simulink model "downlink_4c2t"  (Simulink 8.7)
settings: Solver=VariableStepDiscrete  StartTime=0.0  StopTime=DUC_LINEUP_param.endTime  RelTol=1e-3
PreLoadFcn:
  | % Run the setup script when the model is opened
  | setup_downlink_4c2t;
InitFcn:
  | % Run the setup script again just before the
  | % model is run, so that any updates made
  | % after opening are applied.
  | setup_downlink_4c2t;
  | 
  | %% DSPBuilder Start
  | alt_dspbuilder_update_model(bdroot)
  | %% DSPBuilder End
values from neighbouring files (symbols this model uses):
  LUTS_DPD_CLIP =     [downlink_4c2t_dpd_clip.mat]
  PulsExtention = 128    [setup_downlink_4c2t.m]
  StartAddress1 = Iter1_Param.BaseAddr + 3200    [setup_downlink_4c2t.m]
  StartAddress2 = StartAddress1+1024    [setup_downlink_4c2t.m]
  win = [w(1:PulsExtention) ones(1,Iter0_Param.pulseLen) w(PulsExtention+1:end)]    [setup_downlink_4c2t.m]
undefined symbols (not defined in the file or in its folder): AdvDSPBChannelOutDisplay, AdvDSPBDMemDisplay, dpoly, dspba_ChannelInVis, dspba_ChannelOutVis, dspba_internal_get_channel_ports, dspba_internal_get_demux_ports, DUC_LINEUP_param, evalAionMaskParam, iq_width, Iter0_Param, latency, primtype, REG, UseDontCare, value
undefined symbols (not defined in the file): cfr0_id, cfr_Params0, cfr_Params1, clock_rate, REG_dut_id_addr
libraries: DSPBAPrim x1438, DSPBAControl x77, DSPBAModelBus x71, DSPBABase x40, downlink_4c2t_foldingcfr_3firs_lib x26, DSPBAUtilities x8, downlink_4c2t_lib x4, downlink_4c2t_cordic_lib x2, downlink_4c2t_dpd_clipper x2, DSPBAFilters x2, DSPBAWaveformSynth x2, downlink_4c2t_lduc_lib x1
(part 2 of 17)

== system downlink_4c2t/DUT/COMPLEX_REAL ==
  a1 : Inport
  v : Inport  Port=2
  c : Inport  Port=3
  ChannelIn : DSPBAPrim/ChannelIn  primtype=channelin  nInputs=dspba_internal_get_channel_ports(gcb)  nOutputs=dspba_internal_get_channel_ports(gcb)  omode=Inherit via internal rule  otype=sfix(16)  scale=2^-15  rndmethod=Unbiased  factor=1  satmethod=Symmetric  shift_vec=[0 1 2 -1]  value=1  inPortNames=['v'; 'c'; '0'; '1'; '2'; '3'; '4'; '5'; '6'; '7'; '8'; '9'; 'A'; 'B'; 'D'; 'E'; 'F'; 'G'; 'H'; 'I'; 'J'; 'K'; 'L'; 'M'; 'N'; 'O'; 'P'; 'Q'; 'R'; 'S'; 'T'; 'U'; 'W'; 'X'; 'Y'; 'Z']  outPortNames=['v'; 'c'; '0'; '1'; '2'; '3'; '4'; '5'; '6'; '7'; '8'; '9'; 'A'; 'B'; 'D'; 'E'; 'F'; 'G'; 'H'; 'I'; 'J'; 'K'; 'L'; 'M'; 'N'; 'O'; 'P'; 'Q'; 'R'; 'S'; 'T'; 'U'; 'W'; 'X'; 'Y'; 'Z']  dspbaimage=dspba_prim.jpg  text=fprintf('In');  style=Optimised  dataSignals=1  foldingEnabled=off  channels=1  sampleRate=200  packetBeginPresent=off  packetBeginEnabled=off  visibilities=dspba_ChannelInVis(gcb)  latencyCorrection=0  version=20141013
  ChannelOut : DSPBAPrim/ChannelOut  primtype=channelout  nInputs=dspba_internal_get_channel_ports(gcb)  nOutputs=dspba_internal_get_channel_ports(gcb)  omode=Inherit via internal rule  otype=sfix(16)  scale=2^-15  rndmethod=Unbiased  factor=1  satmethod=Symmetric  shift_vec=[0 1 2 -1]  value=4  inPortNames=['v'; 'c'; '0'; '1'; '2'; '3'; '4'; '5'; '6'; '7'; '8'; '9'; 'A'; 'B'; 'D'; 'E'; 'F'; 'G'; 'H'; 'I'; 'J'; 'K'; 'L'; 'M'; 'N'; 'O'; 'P'; 'Q'; 'R'; 'S'; 'T'; 'U'; 'W'; 'X'; 'Y'; 'Z']  outPortNames=['v'; 'c'; '0'; '1'; '2'; '3'; '4'; '5'; '6'; '7'; '8'; '9'; 'A'; 'B'; 'D'; 'E'; 'F'; 'G'; 'H'; 'I'; 'J'; 'K'; 'L'; 'M'; 'N'; 'O'; 'P'; 'Q'; 'R'; 'S'; 'T'; 'U'; 'W'; 'X'; 'Y'; 'Z']  dspbaimage=dspba_prim.jpg  text=fprintf('Out%s', AdvDSPBChannelOutDisplay(latency));  style=Optimised  dataSignals=4  foldingEnabled=off  channels=1  sampleRate=200  packetBeginPresent=off  packetBeginEnabled=off  visibilities=dspba_ChannelOutVis(gcb)  latency=0  latencyCorrection=0  version=20141013
  Complex to Real-Imag : ComplexToRealImag
  Complex to Real-Imag1 : ComplexToRealImag
  Const : DSPBAPrim/Const  primtype=const  nInputs=0  nOutputs=1  omode=Inherit via internal rule  otype=sfix(16)  scale=2^-15  rndmethod=Unbiased  factor=1  satmethod=Symmetric  shift_vec=[0 1 2 -1]  value=0  inPortNames=['+'; '+';]  outPortNames=[' ']  dspbaimage=dspba_prim.jpg  text=fprintf('%s', num2str(value));  style=Optimised  visibilities=8 + 1024  floatPrecision=float32_m23  version=20120820
  Demux4 : Demux  Outputs=2
  LocalThreshold : DSPBABase/LocalThreshold  margin=DUC_LINEUP_param.ClockMargin  delayRegOrRAMThresholdBits=-1  MediumDualMemThresholdBits=-1  LargeDualMemThresholdBits=-1  hardMultiplierThresholdLuts=-1  complexMultKaratsuba=off  version=0
  Mux : Mux
  SynthesisInfo : DSPBAPrim/SynthesisInfo  primtype=synthinfo  nInputs=0  nOutputs=0  omode=Inherit via internal rule  otype=sfix(16)  scale=2^-15  rndmethod=Truncate  factor=1  satmethod=Symmetric  shift_vec=[0 1 2 -1]  value=99  inPortNames=[' '; ' ';]  outPortNames=[' ']  dspbaimage=dspba_prim_ctrl.jpg  text=fprintf('Style=%s', style);  style=Scheduled  visibilities=2^15+2^17+2^18+2^19  constraintInUse=off  constraintRelation=>  constraintLimit=20  bitAccurate=off  version=20150220
  Terminator17 : Terminator
  q1 : Outport
  q_v : Outport  Port=2
  q_c : Outport  Port=3
  wires:
  ChannelIn/2 -> Terminator17/1
  Const/1 -> ChannelOut/2
  ChannelIn/1 -> ChannelOut/1
  ChannelIn/3 -> Demux4/1
  ChannelOut/2 -> q_c/1
  ChannelOut/1 -> q_v/1
  c/1 -> ChannelIn/2
  v/1 -> ChannelIn/1
  a1/1 -> ChannelIn/3
  Demux4/1 -> Complex to Real-Imag/1
  Demux4/2 -> Complex to Real-Imag1/1
  Complex to Real-Imag/1 -> ChannelOut/3
  Complex to Real-Imag/2 -> ChannelOut/4
  Complex to Real-Imag1/1 -> ChannelOut/5
  Complex to Real-Imag1/2 -> ChannelOut/6
  ChannelOut/3 -> Mux/1
  ChannelOut/4 -> Mux/2
  Mux/1 -> q1/1
  ChannelOut/5 -> Mux/3
  ChannelOut/6 -> Mux/4

== system downlink_4c2t/DUT/DPD ==
  dpd_ant1_data : Inport
  dpd_ant2_data : Inport  Port=2
  sink_valid : Inport  Port=3
  sink_channel : Inport  Port=4
  Const{1..6} (6 alike) : DSPBAPrim/Const  primtype=const  nInputs=0  nOutputs=1  omode=Inherit via internal rule  otype=sfix(16)  scale=2^-15  rndmethod=Unbiased  factor=1  satmethod=Symmetric  shift_vec=[0 1 2 -1]  value=0  inPortNames=['+'; '+';]  outPortNames=[' ']  dspbaimage=dspba_prim.jpg  text=fprintf('%s', num2str(value));  style=Optimised  visibilities=8 + 1024  floatPrecision=float32_m23  version=20120820
  DPD_ANT1 : Subsystem
  DPD_ANT2 : Subsystem
  Terminator{,1..3} (4 alike) : Terminator
  complex_real_converter : Subsystem
  complex_real_converter1 : Subsystem
  source_data : Outport
  source_valid : Outport  Port=2
  source_channel : Outport  Port=3
  source_data1 : Outport  Port=4
  source_valid1 : Outport  Port=5
  source_channel1 : Outport  Port=6
  wires:
  DPD_ANT1/1(v) -> source_valid/1
  DPD_ANT1/2(c) -> source_channel/1
  Const5/1 -> DPD_ANT1/4(sop)
  Const3/1 -> DPD_ANT1/5(eop)
  Const1/1 -> DPD_ANT1/6(Arb)
  DPD_ANT1/4(sop_out) -> Terminator/1
  DPD_ANT1/5(eop_out) -> Terminator1/1
  DPD_ANT2/2(c) -> source_channel1/1
  Const6/1 -> DPD_ANT2/4(sop)
  Const4/1 -> DPD_ANT2/5(eop)
  Const2/1 -> DPD_ANT2/6(Arb)
  DPD_ANT2/4(sop_out) -> Terminator2/1
  DPD_ANT2/5(eop_out) -> Terminator3/1
  sink_channel/1 -> DPD_ANT2/2(channel), DPD_ANT1/2(channel)
  sink_valid/1 -> DPD_ANT2/1(valid), DPD_ANT1/1(valid)
  DPD_ANT2/1(v) -> source_valid1/1
  dpd_ant1_data/1 -> DPD_ANT1/3(xr)
  dpd_ant2_data/1 -> DPD_ANT2/3(xr)
  DPD_ANT1/3(zr) -> complex_real_converter/1(In1)
  complex_real_converter/1(Out1) -> source_data/1
  DPD_ANT2/3(zr) -> complex_real_converter1/1(In1)
  complex_real_converter1/1(Out1) -> source_data1/1

== system downlink_4c2t/DUT/DPD1_CLIPPER ==
  "data " : Inport
  valid : Inport  Port=2
  channel : Inport  Port=3
  scale_bit : Inport  Port=4
  Demux : Demux  Outputs=2
  Scale : DSPBABase/Scale  otype=sfix(16)  scale=2^-15  rndmethod=Unbiased  factor=1  satmethod=Symmetric  shift_vec=[0 1]  latency=9  wideSimulation=off  version=20130807
  Subsystem : Subsystem
  Terminator : Terminator
  bit_combine : downlink_4c2t_dpd_clipper/DPD_CLIPER/Subsystem/complex_real_converter
  DATA_Out : Outport
  Valid_Out : Outport  Port=2
  Chann_Out : Outport  Port=3
  wires:
  bit_combine/1 -> DATA_Out/1
  Scale/1 -> Demux/1
  Demux/1 -> bit_combine/1
  Demux/2 -> bit_combine/2
  Scale/2 -> Valid_Out/1
  Scale/3 -> Chann_Out/1
  scale_bit/1 -> Scale/4
  Scale/4 -> Terminator/1
  Subsystem/1("data_out ") -> Scale/1
  Subsystem/2(valid_out) -> Scale/2
  Subsystem/3(channel_out) -> Scale/3
  "data "/1 -> Subsystem/1(data 1)
  valid/1 -> Subsystem/2(valid1)
  channel/1 -> Subsystem/3(channel1)

== system downlink_4c2t/DUT/DPD2_CLIPPER ==
  "data " : Inport
  valid : Inport  Port=2
  channel : Inport  Port=3
  scale_bit : Inport  Port=4
  Demux : Demux  Outputs=2
  Scale : DSPBABase/Scale  otype=sfix(16)  scale=2^-15  rndmethod=Unbiased  factor=1  satmethod=Symmetric  shift_vec=[0 1]  latency=9  wideSimulation=off  version=20130807
  Subsystem : Subsystem
  Terminator : Terminator
  bit_combine : downlink_4c2t_dpd_clipper/DPD_CLIPER/Subsystem/complex_real_converter
  DATA_Out : Outport
  Valid_Out : Outport  Port=2
  Chann_Out : Outport  Port=3
  wires:
  channel/1 -> Subsystem/3(channel1)
  valid/1 -> Subsystem/2(valid1)
  "data "/1 -> Subsystem/1(data 1)
  Subsystem/3(channel_out) -> Scale/3
  Subsystem/2(valid_out) -> Scale/2
  Subsystem/1("data_out ") -> Scale/1
  Scale/4 -> Terminator/1
  scale_bit/1 -> Scale/4
  Scale/3 -> Chann_Out/1
  Scale/2 -> Valid_Out/1
  Demux/2 -> bit_combine/2
  Demux/1 -> bit_combine/1
  Scale/1 -> Demux/1
  bit_combine/1 -> DATA_Out/1

== system downlink_4c2t/DUT/DPD_ANT1_IN_rfp ==
  GPOut : DSPBAPrim/GPOut  primtype=gpout  nInputs=evalAionMaskParam(gcb,'value',1)  nOutputs=evalAionMaskParam(gcb,'value',1)  omode=Inherit via internal rule  otype=sfix(16)  scale=2^-15  rndmethod=Unbiased  factor=1  satmethod=Symmetric  shift_vec=[0 1 2 -1]  value=1  inPortNames=[' ' ' ' ' ' ' ' ' ' ' ' ' ' ' ' ' ' ' ' ' ' ' ' ' ' ' ' ' ' ' ' ' ' ' ' ' ' ' ' ' ' ' ' ' ' ' ' ' ' ' ' ' ' ' ' ' ' ' ' ' ' ' ' ' ' ' ' ' ']'  outPortNames=[' ' ' ' ' ' ' ' ' ' ' ' ' ' ' ' ' ' ' ' ' ' ' ' ' ' ' ' ' ' ' ' ' ' ' ' ' ' ' ' ' ' ' ' ' ' ' ' ' ' ' ' ' ' ' ' ' ' ' ' ' ' ' ' ' ' ' ' ' ']'  dspbaimage=dspba_prim.jpg  text=fprintf('GPOut');  style=Optimised  visibilities=1024  latencyCorrection=0  version=20090407
  SynthesisInfo : DSPBAPrim/SynthesisInfo  primtype=synthinfo  nInputs=0  nOutputs=0  omode=Inherit via internal rule  otype=sfix(16)  scale=2^-15  rndmethod=Truncate  factor=1  satmethod=Symmetric  shift_vec=[0 1 2 -1]  value=99  inPortNames=[' '; ' ';]  outPortNames=[' ']  dspbaimage=dspba_prim_ctrl.jpg  text=fprintf('Style=%s', style);  style=Scheduled  visibilities=2^15+2^17+2^18+2^19  constraintInUse=off  constraintRelation=>  constraintLimit=2  bitAccurate=off  version=20150220
  zero_idx1 : DSPBAPrim/Const  primtype=const  nInputs=0  nOutputs=1  omode=boolean  otype=ufix(1)  scale=0  rndmethod=Unbiased  factor=1  satmethod=Symmetric  shift_vec=[0 1 2 -1]  value=1  inPortNames=['+'; '+';]  outPortNames=[' ']  dspbaimage=dspba_prim.jpg  text=fprintf('%s', num2str(value));  style=Optimised  visibilities=8 + 1024  floatPrecision=float32_m23  version=20120820
  Out_RFP : Outport
  wires:
  GPOut/1 -> Out_RFP/1
  zero_idx1/1 -> GPOut/1

== system downlink_4c2t/DUT/DUC_DPD1_OUT_PM ==
  note: I^2 + Q^2
  valid : Inport
  channel : Inport  Port=2
  "data " : Inport  Port=3
  pulse_1msec : Inport  Port=4
  Reg_busy_bit : Inport  Port=5
  Ant1_accumulator : Subsystem
  Ant1_peak_dedector : Subsystem
  BitExtract : DSPBAPrim/BitExtract  primtype=bitextract  nInputs=1  nOutputs=1  omode=Specify via dialog  otype=ufix(32)  scale=2^0  rndmethod=Unbiased  factor=1  satmethod=Symmetric  shift_vec=[0 1 2 -1]  value=0  inPortNames=[' '; ' ';]  outPortNames=[' ']  dspbaimage=dspba_prim.jpg  text=fprintf('..%d', value);  style=Optimised  visibilities=8+1024  version=20090407
  BitExtract1 : DSPBAPrim/BitExtract  primtype=bitextract  nInputs=1  nOutputs=1  omode=Specify via dialog  otype=ufix(32)  scale=2^0  rndmethod=Unbiased  factor=1  satmethod=Symmetric  shift_vec=[0 1 2 -1]  value=32  inPortNames=[' '; ' ';]  outPortNames=[' ']  dspbaimage=dspba_prim.jpg  text=fprintf('..%d', value);  style=Optimised  visibilities=8+1024  version=20090407
  Carr1_Accumulater1 : DSPBAModelBus/RegOut  reg_name=power_meter_param.dpd1_out_acc1_reg_addr  reg_rwmode=Read  reg_msb=31  reg_lsb=0  reg_desc=Description of what is stored in this register  reg_addr=9681  SampleTime=-1  version=20090407
  Carr1_Accumulater2 : DSPBAModelBus/RegOut  reg_name=power_meter_param.dpd1_out_acc2_reg_addr  reg_rwmode=Read  reg_msb=31  reg_lsb=0  reg_desc=Description of what is stored in this register  reg_addr=9682  SampleTime=-1  version=20090407
  Carr1_PD : DSPBAModelBus/RegOut  reg_name=power_meter_param.dpd1_out_pd_address  reg_rwmode=Read  reg_msb=31  reg_lsb=0  reg_desc=Description of what is stored in this register  reg_addr=9680  SampleTime=-1  version=20090407
  Const : DSPBAPrim/Const  primtype=const  nInputs=0  nOutputs=1  omode=Inherit via internal rule  otype=sfix(16)  scale=2^-15  rndmethod=Unbiased  factor=1  satmethod=Symmetric  shift_vec=[0 1 2 -1]  value=0  inPortNames=['+'; '+';]  outPortNames=[' ']  dspbaimage=dspba_prim.jpg  text=fprintf('%s', num2str(value));  style=Optimised  visibilities=8 + 1024  floatPrecision=float32_m23  version=20120820
  Edge_deductor : Subsystem
  Scale : DSPBABase/Scale  otype=sfix(16)  scale=2^-15  rndmethod=Unbiased  factor=1  satmethod=Symmetric  shift_vec=0  latency=6  wideSimulation=off  version=20130807
  Terminator1 : Terminator
  carrier_separation : Subsystem
  wires:
  BitExtract1/1 -> Carr1_Accumulater2/1
  BitExtract/1 -> Carr1_Accumulater1/1
  carrier_separation/3(channel_out) -> Scale/3
  carrier_separation/2(valid_out) -> Scale/2
  pulse_1msec/1 -> carrier_separation/4("1ms_pulse_in ")
  Scale/4 -> Terminator1/1
  "data "/1 -> carrier_separation/3("data ")
  channel/1 -> carrier_separation/2(channel)
  valid/1 -> carrier_separation/1(valid)
  Scale/2 -> Ant1_accumulator/2(valid1), Ant1_peak_dedector/2(valid)
  Scale/3 -> Ant1_accumulator/3(channel1), Ant1_peak_dedector/3(channel)
  Const/1 -> Scale/4
  carrier_separation/1("axc1_data_out ") -> Scale/1
  Scale/1 -> Ant1_accumulator/1(data), Ant1_peak_dedector/1(data_in)
  carrier_separation/4(pulse_1ms_out) -> Ant1_peak_dedector/4(pulse_1ms), Ant1_accumulator/4(pulse_1ms)
  Ant1_peak_dedector/1(Out_data) -> Carr1_PD/1
  Edge_deductor/1(Out1) -> Carr1_Accumulater2/2, Carr1_Accumulater1/2, Carr1_PD/2
  Ant1_peak_dedector/2(pulse_1ms_out) -> Edge_deductor/2(In2)
  Reg_busy_bit/1 -> Edge_deductor/1(In1)
  Ant1_accumulator/1(Out_data) -> BitExtract/1, BitExtract1/1

== system downlink_4c2t/DUT/DUC_DPD2_OUT_PM ==
  note: I^2 + Q^2
  valid : Inport
  channel : Inport  Port=2
  "data " : Inport  Port=3
  pulse_1msec : Inport  Port=4
  Reg_busy_bit : Inport  Port=5
  Ant1_accumulator : Subsystem
  Ant1_peak_dedector : Subsystem
  BitExtract : DSPBAPrim/BitExtract  primtype=bitextract  nInputs=1  nOutputs=1  omode=Specify via dialog  otype=ufix(32)  scale=2^0  rndmethod=Unbiased  factor=1  satmethod=Symmetric  shift_vec=[0 1 2 -1]  value=0  inPortNames=[' '; ' ';]  outPortNames=[' ']  dspbaimage=dspba_prim.jpg  text=fprintf('..%d', value);  style=Optimised  visibilities=8+1024  version=20090407
  BitExtract1 : DSPBAPrim/BitExtract  primtype=bitextract  nInputs=1  nOutputs=1  omode=Specify via dialog  otype=ufix(32)  scale=2^0  rndmethod=Unbiased  factor=1  satmethod=Symmetric  shift_vec=[0 1 2 -1]  value=32  inPortNames=[' '; ' ';]  outPortNames=[' ']  dspbaimage=dspba_prim.jpg  text=fprintf('..%d', value);  style=Optimised  visibilities=8+1024  version=20090407
  Carr1_Accumulater1 : DSPBAModelBus/RegOut  reg_name=power_meter_param.dpd2_out_acc1_reg_addr  reg_rwmode=Read  reg_msb=31  reg_lsb=0  reg_desc=Description of what is stored in this register  reg_addr=9684  SampleTime=-1  version=20090407
  Carr1_Accumulater2 : DSPBAModelBus/RegOut  reg_name=power_meter_param.dpd2_out_acc2_reg_addr  reg_rwmode=Read  reg_msb=31  reg_lsb=0  reg_desc=Description of what is stored in this register  reg_addr=9685  SampleTime=-1  version=20090407
  Carr1_PD : DSPBAModelBus/RegOut  reg_name=power_meter_param.dpd2_out_pd_address  reg_rwmode=Read  reg_msb=31  reg_lsb=0  reg_desc=Description of what is stored in this register  reg_addr=9683  SampleTime=-1  version=20090407
  Const : DSPBAPrim/Const  primtype=const  nInputs=0  nOutputs=1  omode=Inherit via internal rule  otype=sfix(16)  scale=2^-15  rndmethod=Unbiased  factor=1  satmethod=Symmetric  shift_vec=[0 1 2 -1]  value=0  inPortNames=['+'; '+';]  outPortNames=[' ']  dspbaimage=dspba_prim.jpg  text=fprintf('%s', num2str(value));  style=Optimised  visibilities=8 + 1024  floatPrecision=float32_m23  version=20120820
  Edge_deductor : Subsystem
  Scale : DSPBABase/Scale  otype=sfix(16)  scale=2^-15  rndmethod=Unbiased  factor=1  satmethod=Symmetric  shift_vec=0  latency=6  wideSimulation=off  version=20130807
  Terminator1 : Terminator
  carrier_separation : Subsystem
  wires:
  Reg_busy_bit/1 -> Edge_deductor/1(In1)
  Ant1_peak_dedector/2(pulse_1ms_out) -> Edge_deductor/2(In2)
  Edge_deductor/1(Out1) -> Carr1_PD/2, Carr1_Accumulater1/2, Carr1_Accumulater2/2
  Ant1_peak_dedector/1(Out_data) -> Carr1_PD/1
  carrier_separation/4(pulse_1ms_out) -> Ant1_accumulator/4(pulse_1ms), Ant1_peak_dedector/4(pulse_1ms)
  Scale/1 -> Ant1_peak_dedector/1(data_in), Ant1_accumulator/1(data)
  carrier_separation/1("axc1_data_out ") -> Scale/1
  Const/1 -> Scale/4
  Scale/3 -> Ant1_peak_dedector/3(channel), Ant1_accumulator/3(channel1)
  Scale/2 -> Ant1_peak_dedector/2(valid), Ant1_accumulator/2(valid1)
  valid/1 -> carrier_separation/1(valid)
  channel/1 -> carrier_separation/2(channel)
  "data "/1 -> carrier_separation/3("data ")
  Scale/4 -> Terminator1/1
  pulse_1msec/1 -> carrier_separation/4("1ms_pulse_in ")
  carrier_separation/2(valid_out) -> Scale/2
  carrier_separation/3(channel_out) -> Scale/3
  BitExtract/1 -> Carr1_Accumulater1/1
  BitExtract1/1 -> Carr1_Accumulater2/1
  Ant1_accumulator/1(Out_data) -> BitExtract/1, BitExtract1/1

== system downlink_4c2t/DUT/DUC_DPD_IN_PM ==
  note: I^2 + Q^2
  valid : Inport
  channel : Inport  Port=2
  "data " : Inport  Port=3
  pulse_1msec : Inport  Port=4
  Reg_busy_bit : Inport  Port=5
  Ant1_accumulator : Subsystem
  Ant1_peak_dedector : Subsystem
  Ant2_accumulator : Subsystem
  Ant2_peak_dedector : Subsystem
  BitExtract : DSPBAPrim/BitExtract  primtype=bitextract  nInputs=1  nOutputs=1  omode=Specify via dialog  otype=ufix(32)  scale=2^0  rndmethod=Unbiased  factor=1  satmethod=Symmetric  shift_vec=[0 1 2 -1]  value=0  inPortNames=[' '; ' ';]  outPortNames=[' ']  dspbaimage=dspba_prim.jpg  text=fprintf('..%d', value);  style=Optimised  visibilities=8+1024  version=20090407
  BitExtract1 : DSPBAPrim/BitExtract  primtype=bitextract  nInputs=1  nOutputs=1  omode=Specify via dialog  otype=ufix(32)  scale=2^0  rndmethod=Unbiased  factor=1  satmethod=Symmetric  shift_vec=[0 1 2 -1]  value=32  inPortNames=[' '; ' ';]  outPortNames=[' ']  dspbaimage=dspba_prim.jpg  text=fprintf('..%d', value);  style=Optimised  visibilities=8+1024  version=20090407
  BitExtract2 : DSPBAPrim/BitExtract  primtype=bitextract  nInputs=1  nOutputs=1  omode=Specify via dialog  otype=ufix(32)  scale=2^0  rndmethod=Unbiased  factor=1  satmethod=Symmetric  shift_vec=[0 1 2 -1]  value=0  inPortNames=[' '; ' ';]  outPortNames=[' ']  dspbaimage=dspba_prim.jpg  text=fprintf('..%d', value);  style=Optimised  visibilities=8+1024  version=20090407
  BitExtract3 : DSPBAPrim/BitExtract  primtype=bitextract  nInputs=1  nOutputs=1  omode=Specify via dialog  otype=ufix(32)  scale=2^0  rndmethod=Unbiased  factor=1  satmethod=Symmetric  shift_vec=[0 1 2 -1]  value=32  inPortNames=[' '; ' ';]  outPortNames=[' ']  dspbaimage=dspba_prim.jpg  text=fprintf('..%d', value);  style=Optimised  visibilities=8+1024  version=20090407
  Carr1_Accumulater1 : DSPBAModelBus/RegOut  reg_name=power_meter_param.dpd1_in_acc1_reg_addr  reg_rwmode=Read  reg_msb=31  reg_lsb=0  reg_desc=Description of what is stored in this register  reg_addr=9676  SampleTime=-1  version=20090407
  Carr1_Accumulater2 : DSPBAModelBus/RegOut  reg_name=power_meter_param.dpd1_in_acc2_reg_addr  reg_rwmode=Read  reg_msb=31  reg_lsb=0  reg_desc=Description of what is stored in this register  reg_addr=9677  SampleTime=-1  version=20090407
  Carr1_PD : DSPBAModelBus/RegOut  reg_name=power_meter_param.dpd1_in_pd_address  reg_rwmode=Read  reg_msb=31  reg_lsb=0  reg_desc=Description of what is stored in this register  reg_addr=9674  SampleTime=-1  version=20090407
  Carr2_Accumulater1 : DSPBAModelBus/RegOut  reg_name=power_meter_param.dpd2_in_acc1_reg_addr  reg_rwmode=Read  reg_msb=31  reg_lsb=0  reg_desc=Description of what is stored in this register  reg_addr=9678  SampleTime=-1  version=20090407
  Carr2_Accumulater2 : DSPBAModelBus/RegOut  reg_name=power_meter_param.dpd2_in_acc2_reg_addr  reg_rwmode=Read  reg_msb=31  reg_lsb=0  reg_desc=Description of what is stored in this register  reg_addr=9679  SampleTime=-1  version=20090407
  Carr2_PD : DSPBAModelBus/RegOut  reg_name=power_meter_param.dpd2_in_pd_address  reg_rwmode=Read  reg_msb=31  reg_lsb=0  reg_desc=Description of what is stored in this register  reg_addr=9675  SampleTime=-1  version=20090407
  Const : DSPBAPrim/Const  primtype=const  nInputs=0  nOutputs=1  omode=Inherit via internal rule  otype=sfix(16)  scale=2^-15  rndmethod=Unbiased  factor=1  satmethod=Symmetric  shift_vec=[0 1 2 -1]  value=0  inPortNames=['+'; '+';]  outPortNames=[' ']  dspbaimage=dspba_prim.jpg  text=fprintf('%s', num2str(value));  style=Optimised  visibilities=8 + 1024  floatPrecision=float32_m23  version=20120820
  Demux : Demux  Outputs=2
  Edge_deductor : Subsystem
  Edge_deductor1 : Subsystem
  Mux : Mux  Inputs=2
  Scale : DSPBABase/Scale  otype=sfix(16)  scale=2^-15  rndmethod=Unbiased  factor=1  satmethod=Symmetric  shift_vec=0  latency=6  wideSimulation=off  version=20130807
  Terminator1 : Terminator
  carrier_separation : Subsystem
  wires:
  BitExtract3/1 -> Carr2_Accumulater2/1
  BitExtract2/1 -> Carr2_Accumulater1/1
  BitExtract1/1 -> Carr1_Accumulater2/1
  BitExtract/1 -> Carr1_Accumulater1/1
  carrier_separation/4(channel_out) -> Scale/3
  carrier_separation/3(valid_out) -> Scale/2
  pulse_1msec/1 -> carrier_separation/4("1ms_pulse_in ")
  Scale/4 -> Terminator1/1
  "data "/1 -> carrier_separation/3("data ")
  channel/1 -> carrier_separation/2(channel)
  valid/1 -> carrier_separation/1(valid)
  carrier_separation/1("axc1_data_out ") -> Mux/1
  carrier_separation/2(axc2_valid_out) -> Mux/2
  Mux/1 -> Scale/1
  Scale/1 -> Demux/1
  Const/1 -> Scale/4
  Demux/1 -> Ant1_accumulator/1(data), Ant1_peak_dedector/1(data_in)
  Demux/2 -> Ant2_accumulator/1(data), Ant2_peak_dedector/1(data_in)
  Scale/2 -> Ant1_peak_dedector/2(valid), Ant1_accumulator/2(valid1), Ant2_peak_dedector/2(valid), Ant2_accumulator/2(valid1)
  Scale/3 -> Ant2_peak_dedector/3(channel), Ant2_accumulator/3(channel1), Ant1_accumulator/3(channel1), Ant1_peak_dedector/3(channel)
  carrier_separation/5(pulse_1ms_out) -> Ant2_peak_dedector/4(pulse_1ms), Ant1_accumulator/4(pulse_1ms), Ant1_peak_dedector/4(pulse_1ms), Ant2_accumulator/4(pulse_1ms)
  Ant1_peak_dedector/1(Out_data) -> Carr1_PD/1
  Ant1_peak_dedector/2(pulse_1ms_out) -> Edge_deductor1/2(In2)
  Edge_deductor1/1(Out1) -> Carr1_Accumulater1/2, Carr1_Accumulater2/2, Carr1_PD/2
  Ant1_accumulator/1(Out_data) -> BitExtract/1, BitExtract1/1
  Ant2_peak_dedector/2(pulse_1ms_out) -> Edge_deductor/2(In2)
  Edge_deductor/1(Out1) -> Carr2_Accumulater1/2, Carr2_Accumulater2/2, Carr2_PD/2
  Ant2_peak_dedector/1(Out_data) -> Carr2_PD/1
  Ant2_accumulator/1(Out_data) -> BitExtract2/1, BitExtract3/1
  Reg_busy_bit/1 -> Edge_deductor1/1(In1), Edge_deductor/1(In1)

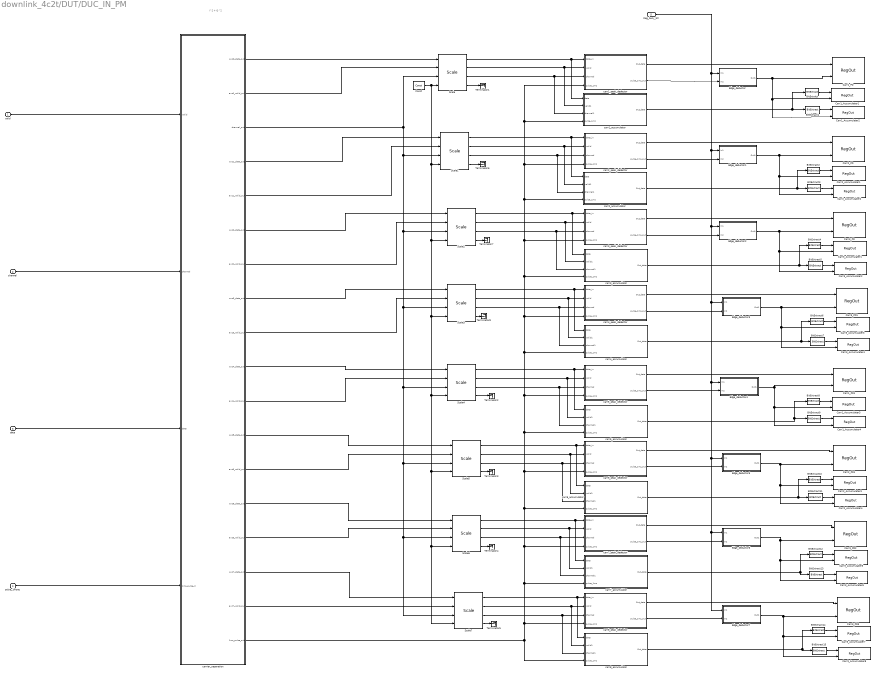
== system downlink_4c2t/DUT/DUC_IN_PM ==
  note: I^2 + Q^2
  valid : Inport
  channel : Inport  Port=2
  "data " : Inport  Port=3
  pulse_1msec : Inport  Port=4
  Reg_busy_bit : Inport  Port=5
  BitExtract{,2,4,6,8,10,12,14} (8 alike) : DSPBAPrim/BitExtract  primtype=bitextract  nInputs=1  nOutputs=1  omode=Specify via dialog  otype=ufix(32)  scale=2^0  rndmethod=Unbiased  factor=1  satmethod=Symmetric  shift_vec=[0 1 2 -1]  value=0  inPortNames=[' '; ' ';]  outPortNames=[' ']  dspbaimage=dspba_prim.jpg  text=fprintf('..%d', value);  style=Optimised  visibilities=8+1024  version=20090407
  BitExtract{1,3,5,7,9,11,13,15} (8 alike) : DSPBAPrim/BitExtract  primtype=bitextract  nInputs=1  nOutputs=1  omode=Specify via dialog  otype=ufix(32)  scale=2^0  rndmethod=Unbiased  factor=1  satmethod=Symmetric  shift_vec=[0 1 2 -1]  value=32  inPortNames=[' '; ' ';]  outPortNames=[' ']  dspbaimage=dspba_prim.jpg  text=fprintf('..%d', value);  style=Optimised  visibilities=8+1024  version=20090407
  Carr1_Accumulater1 : DSPBAModelBus/RegOut  reg_name=power_meter_param.carr1_acc1_reg_addr  reg_rwmode=Read  reg_msb=31  reg_lsb=0  reg_desc=Description of what is stored in this register  reg_addr=9652  SampleTime=-1  version=20090407
  Carr1_Accumulater2 : DSPBAModelBus/RegOut  reg_name=power_meter_param.carr1_acc2_reg_addr  reg_rwmode=Read  reg_msb=31  reg_lsb=0  reg_desc=Description of what is stored in this register  reg_addr=9653  SampleTime=-1  version=20090407
  Carr1_Accumulater3 : DSPBAModelBus/RegOut  reg_name=power_meter_param.carr5_acc1_reg_addr  reg_rwmode=Read  reg_msb=31  reg_lsb=0  reg_desc=Description of what is stored in this register  reg_addr=9660  SampleTime=-1  version=20090407
  Carr1_Accumulater4 : DSPBAModelBus/RegOut  reg_name=power_meter_param.carr5_acc2_reg_addr  reg_rwmode=Read  reg_msb=31  reg_lsb=0  reg_desc=Description of what is stored in this register  reg_addr=9661  SampleTime=-1  version=20090407
  Carr1_PD : DSPBAModelBus/RegOut  reg_name=power_meter_param.carr1_pd_address  reg_rwmode=Read  reg_msb=31  reg_lsb=0  reg_desc=Description of what is stored in this register  reg_addr=9644  SampleTime=-1  version=20090407
  Carr1_PD1 : DSPBAModelBus/RegOut  reg_name=power_meter_param.carr5_pd_address  reg_rwmode=Read  reg_msb=31  reg_lsb=0  reg_desc=Description of what is stored in this register  reg_addr=9648  SampleTime=-1  version=20090407
  Carr2_Accumulater1 : DSPBAModelBus/RegOut  reg_name=power_meter_param.carr2_acc1_reg_addr  reg_rwmode=Read  reg_msb=31  reg_lsb=0  reg_desc=Description of what is stored in this register  reg_addr=9654  SampleTime=-1  version=20090407
  Carr2_Accumulater2 : DSPBAModelBus/RegOut  reg_name=power_meter_param.carr2_acc2_reg_addr  reg_rwmode=Read  reg_msb=31  reg_lsb=0  reg_desc=Description of what is stored in this register  reg_addr=9655  SampleTime=-1  version=20090407
  Carr2_Accumulater3 : DSPBAModelBus/RegOut  reg_name=power_meter_param.carr6_acc1_reg_addr  reg_rwmode=Read  reg_msb=31  reg_lsb=0  reg_desc=Description of what is stored in this register  reg_addr=9662  SampleTime=-1  version=20090407
  Carr2_Accumulater4 : DSPBAModelBus/RegOut  reg_name=power_meter_param.carr6_acc2_reg_addr  reg_rwmode=Read  reg_msb=31  reg_lsb=0  reg_desc=Description of what is stored in this register  reg_addr=9663  SampleTime=-1  version=20090407
  Carr2_PD : DSPBAModelBus/RegOut  reg_name=power_meter_param.carr2_pd_address  reg_rwmode=Read  reg_msb=31  reg_lsb=0  reg_desc=Description of what is stored in this register  reg_addr=9645  SampleTime=-1  version=20090407
  Carr2_PD1 : DSPBAModelBus/RegOut  reg_name=power_meter_param.carr6_pd_address  reg_rwmode=Read  reg_msb=31  reg_lsb=0  reg_desc=Description of what is stored in this register  reg_addr=9649  SampleTime=-1  version=20090407
  Carr3_Accumulater1 : DSPBAModelBus/RegOut  reg_name=power_meter_param.carr3_acc1_reg_addr  reg_rwmode=Read  reg_msb=31  reg_lsb=0  reg_desc=Description of what is stored in this register  reg_addr=9656  SampleTime=-1  version=20090407
  Carr3_Accumulater2 : DSPBAModelBus/RegOut  reg_name=power_meter_param.carr3_acc2_reg_addr  reg_rwmode=Read  reg_msb=31  reg_lsb=0  reg_desc=Description of what is stored in this register  reg_addr=9657  SampleTime=-1  version=20090407
  Carr3_Accumulater3 : DSPBAModelBus/RegOut  reg_name=power_meter_param.carr4_acc1_reg_addr  reg_rwmode=Read  reg_msb=31  reg_lsb=0  reg_desc=Description of what is stored in this register  reg_addr=9658  SampleTime=-1  version=20090407
  Carr3_Accumulater4 : DSPBAModelBus/RegOut  reg_name=power_meter_param.carr4_acc2_reg_addr  reg_rwmode=Read  reg_msb=31  reg_lsb=0  reg_desc=Description of what is stored in this register  reg_addr=9659  SampleTime=-1  version=20090407
  Carr3_Accumulater5 : DSPBAModelBus/RegOut  reg_name=power_meter_param.carr7_acc1_reg_addr  reg_rwmode=Read  reg_msb=31  reg_lsb=0  reg_desc=Description of what is stored in this register  reg_addr=9664  SampleTime=-1  version=20090407
  Carr3_Accumulater6 : DSPBAModelBus/RegOut  reg_name=power_meter_param.carr7_acc2_reg_addr  reg_rwmode=Read  reg_msb=31  reg_lsb=0  reg_desc=Description of what is stored in this register  reg_addr=9665  SampleTime=-1  version=20090407
  Carr3_Accumulater7 : DSPBAModelBus/RegOut  reg_name=power_meter_param.carr8_acc1_reg_addr  reg_rwmode=Read  reg_msb=31  reg_lsb=0  reg_desc=Description of what is stored in this register  reg_addr=9666  SampleTime=-1  version=20090407
  Carr3_Accumulater8 : DSPBAModelBus/RegOut  reg_name=power_meter_param.carr8_acc2_reg_addr  reg_rwmode=Read  reg_msb=31  reg_lsb=0  reg_desc=Description of what is stored in this register  reg_addr=9667  SampleTime=-1  version=20090407
  Carr3_PD : DSPBAModelBus/RegOut  reg_name=power_meter_param.carr3_pd_address  reg_rwmode=Read  reg_msb=31  reg_lsb=0  reg_desc=Description of what is stored in this register  reg_addr=9646  SampleTime=-1  version=20090407
  Carr3_PD1 : DSPBAModelBus/RegOut  reg_name=power_meter_param.carr4_pd_address  reg_rwmode=Read  reg_msb=31  reg_lsb=0  reg_desc=Description of what is stored in this register  reg_addr=9647  SampleTime=-1  version=20090407
  Carr3_PD2 : DSPBAModelBus/RegOut  reg_name=power_meter_param.carr7_pd_address  reg_rwmode=Read  reg_msb=31  reg_lsb=0  reg_desc=Description of what is stored in this register  reg_addr=9650  SampleTime=-1  version=20090407
  Carr3_PD3 : DSPBAModelBus/RegOut  reg_name=power_meter_param.carr8_pd_address  reg_rwmode=Read  reg_msb=31  reg_lsb=0  reg_desc=Description of what is stored in this register  reg_addr=9651  SampleTime=-1  version=20090407
  Const : DSPBAPrim/Const  primtype=const  nInputs=0  nOutputs=1  omode=Inherit via internal rule  otype=sfix(16)  scale=2^-15  rndmethod=Unbiased  factor=1  satmethod=Symmetric  shift_vec=[0 1 2 -1]  value=0  inPortNames=['+'; '+';]  outPortNames=[' ']  dspbaimage=dspba_prim.jpg  text=fprintf('%s', num2str(value));  style=Optimised  visibilities=8 + 1024  floatPrecision=float32_m23  version=20120820
  Edge_deductor : Subsystem
  Edge_deductor1 : Subsystem
  Edge_deductor2 : Subsystem
  Edge_deductor3 : Subsystem
  Edge_deductor4 : Subsystem
  Edge_deductor5 : Subsystem
  Edge_deductor6 : Subsystem
  Edge_deductor7 : Subsystem
  Scale{,1..7} (8 alike) : DSPBABase/Scale  otype=sfix(16)  scale=2^-15  rndmethod=Unbiased  factor=1  satmethod=Symmetric  shift_vec=0  latency=6  wideSimulation=off  version=20130807
  Terminator{1..8} (8 alike) : Terminator
  carr1_accumulator : Subsystem
  carr1_peak_dedector : Subsystem
  carr2_accumulator : Subsystem
  carr2_peak_dedector : Subsystem
  carr3_accumulator : Subsystem
  carr3_peak_dedector : Subsystem
  carr4_accumulator : Subsystem
  carr4_peak_dedector : Subsystem
  carr5_accumulator : Subsystem
  carr5_peak_dedector : Subsystem
  carr6_accumulator : Subsystem
  carr6_peak_dedector : Subsystem
  carr7_accumulator : Subsystem
  carr7_peak_dedector : Subsystem
  carr8_accumulator : Subsystem
  carr8_peak_dedector : Subsystem
  carrier_separation : Subsystem
  wires:
  valid/1 -> carrier_separation/1(valid)
  channel/1 -> carrier_separation/2(channel)
  "data "/1 -> carrier_separation/3("data ")
  Scale/4 -> Terminator1/1
  pulse_1msec/1 -> carrier_separation/4("1ms_pulse_in ")
  Scale4/4 -> Terminator2/1
  Scale5/4 -> Terminator3/1
  Scale6/4 -> Terminator4/1
  Scale7/4 -> Terminator5/1
  Scale3/4 -> Terminator8/1
  Scale2/4 -> Terminator7/1
  Scale1/4 -> Terminator6/1
  BitExtract/1 -> Carr1_Accumulater1/1
  BitExtract1/1 -> Carr1_Accumulater2/1
  carr1_accumulator/1(Out_data) -> BitExtract/1, BitExtract1/1
  BitExtract2/1 -> Carr2_Accumulater1/1
  BitExtract3/1 -> Carr2_Accumulater2/1
  BitExtract4/1 -> Carr3_Accumulater1/1
  BitExtract5/1 -> Carr3_Accumulater2/1
  carr1_peak_dedector/2(pulse_1ms_out) -> Edge_deductor/2(In2)
  Reg_busy_bit/1 -> Edge_deductor/1(In1), Edge_deductor1/1(In1), Edge_deductor2/1(In1), Edge_deductor3/1(In1), Edge_deductor4/1(In1), Edge_deductor5/1(In1), Edge_deductor7/1(In1), Edge_deductor6/1(In1)
  Edge_deductor/1(Out1) -> Carr1_Accumulater2/2, Carr1_Accumulater1/2, Carr1_PD/2
  Scale/2 -> carr1_accumulator/2(valid1), carr1_peak_dedector/2(valid)
  Scale/3 -> carr1_accumulator/3(channel1), carr1_peak_dedector/3(channel)
  Scale/1 -> carr1_accumulator/1(data), carr1_peak_dedector/1(data_in)
  Scale1/1 -> carr2_accumulator/1(data), carr2_peak_dedector/1(data_in)
  Scale1/2 -> carr2_accumulator/2(valid1), carr2_peak_dedector/2(valid)
  Scale1/3 -> carr2_accumulator/3(channel1), carr2_peak_dedector/3(channel)
  Scale2/1 -> carr3_accumulator/1(data), carr3_peak_dedector/1(data_in)
  Scale2/2 -> carr3_accumulator/2(valid1), carr3_peak_dedector/2(valid)
  Scale2/3 -> carr3_accumulator/3(channel1), carr3_peak_dedector/3(channel)
  Scale3/1 -> carr4_accumulator/1(data), carr4_peak_dedector/1(data_in)
  Scale3/2 -> carr4_accumulator/2(valid1), carr4_peak_dedector/2(valid)
  Scale3/3 -> carr4_accumulator/3(channel1), carr4_peak_dedector/3(channel)
  Scale4/1 -> carr5_accumulator/1(data), carr5_peak_dedector/1(data_in)
  Scale4/2 -> carr5_accumulator/2(valid1), carr5_peak_dedector/2(valid)
  Scale4/3 -> carr5_accumulator/3(channel1), carr5_peak_dedector/3(channel)
  carrier_separation/18(1ms_pulse_out) -> carr8_peak_dedector/4(pulse_1ms), carr7_accumulator/4(pulse_1ms), carr6_accumulator/4(pulse_1ms), carr6_peak_dedector/4(pulse_1ms), carr5_accumulator/4(pulse_1ms), carr5_peak_dedector/4(pulse_1ms), carr4_accumulator/4(pulse_1ms), carr4_peak_dedector/4(pulse_1ms), carr2_accumulator/4(pulse_1ms), carr2_peak_dedector/4(pulse_1ms), carr1_accumulator/4(pulse_1ms), carr1_peak_dedector/4(pulse_1ms), carr3_peak_dedector/4(pulse_1ms), carr3_accumulator/4(pulse_1ms), carr7_peak_dedector/4(pulse_1ms), carr8_accumulator/4(pulse_1ms)
  Scale5/1 -> carr6_accumulator/1(data), carr6_peak_dedector/1(data_in)
  Scale5/2 -> carr6_accumulator/2(valid1), carr6_peak_dedector/2(valid)
  Scale5/3 -> carr6_accumulator/3(channel1), carr6_peak_dedector/3(channel)
  Scale6/1 -> carr7_accumulator/1(data), carr7_peak_dedector/1(data_in)
  Scale6/2 -> carr7_accumulator/2(valid1), carr7_peak_dedector/2(valid)
  Scale6/3 -> carr7_accumulator/3(channel1), carr7_peak_dedector/3(channel)
  Scale7/1 -> carr8_accumulator/1(data), carr8_peak_dedector/1(data_in)
  Scale7/2 -> carr8_accumulator/2(valid1), carr8_peak_dedector/2(valid)
  Scale7/3 -> carr8_accumulator/3(channel1), carr8_peak_dedector/3(channel)
  carrier_separation/2(axc0_valid_out) -> Scale/2
  carrier_separation/1("axc0_data_out ") -> Scale/1
  carrier_separation/4(axc1_data_out) -> Scale1/1
  carrier_separation/5(axc1_valid_out) -> Scale1/2
  carrier_separation/3(channel_out) -> Scale/3, Scale1/3, Scale2/3, Scale4/3, Scale7/3, Scale6/3, Scale5/3, Scale3/3
  carrier_separation/6(axc2_data_out) -> Scale2/1
  carrier_separation/7(axc2_valid_out) -> Scale2/2
  carrier_separation/8(axc3_data_out) -> Scale3/1
  carrier_separation/9(axc3_valid_out) -> Scale3/2
  carrier_separation/10(axc4_data_out) -> Scale4/1
  carrier_separation/11(axc4_valid_out) -> Scale4/2
  carrier_separation/12(axc5_data_out) -> Scale5/1
  carrier_separation/13(axc5_valid_out) -> Scale5/2
  carrier_separation/14(axc6_data_out) -> Scale6/1
  carrier_separation/15(axc6_valid_out) -> Scale6/2
  carrier_separation/16(axc7_data_out) -> Scale7/1
  carrier_separation/17(axc7_valid_out) -> Scale7/2
  Const/1 -> Scale/4, Scale1/4, Scale2/4, Scale3/4, Scale6/4, Scale7/4, Scale5/4, Scale4/4
  carr2_peak_dedector/2(pulse_1ms_out) -> Edge_deductor1/2(In2)
  carr2_peak_dedector/1(Out_data) -> Carr2_PD/1
  carr2_accumulator/1(Out_data) -> BitExtract2/1, BitExtract3/1
  Edge_deductor1/1(Out1) -> Carr2_Accumulater1/2, Carr2_Accumulater2/2, Carr2_PD/2
  carr3_peak_dedector/2(pulse_1ms_out) -> Edge_deductor2/2(In2)
  Edge_deductor2/1(Out1) -> Carr3_Accumulater2/2, Carr3_Accumulater1/2, Carr3_PD/2
  carr3_peak_dedector/1(Out_data) -> Carr3_PD/1
  carr3_accumulator/1(Out_data) -> BitExtract4/1, BitExtract5/1
  BitExtract6/1 -> Carr3_Accumulater3/1
  BitExtract7/1 -> Carr3_Accumulater4/1
  carr4_peak_dedector/2(pulse_1ms_out) -> Edge_deductor3/2(In2)
  Edge_deductor3/1(Out1) -> Carr3_PD1/2, Carr3_Accumulater3/2, Carr3_Accumulater4/2
  carr4_peak_dedector/1(Out_data) -> Carr3_PD1/1
  carr4_accumulator/1(Out_data) -> BitExtract7/1, BitExtract6/1
  BitExtract8/1 -> Carr1_Accumulater3/1
  BitExtract9/1 -> Carr1_Accumulater4/1
  carr5_peak_dedector/1(Out_data) -> Carr1_PD1/1
  carr5_accumulator/1(Out_data) -> BitExtract9/1, BitExtract8/1
  BitExtract10/1 -> Carr2_Accumulater3/1
  BitExtract11/1 -> Carr2_Accumulater4/1
  BitExtract12/1 -> Carr3_Accumulater5/1
  BitExtract13/1 -> Carr3_Accumulater6/1
  carr5_peak_dedector/2(pulse_1ms_out) -> Edge_deductor4/2(In2)
  Edge_deductor4/1(Out1) -> Carr1_PD1/2, Carr1_Accumulater3/2, Carr1_Accumulater4/2
  carr6_peak_dedector/2(pulse_1ms_out) -> Edge_deductor5/2(In2)
  carr6_peak_dedector/1(Out_data) -> Carr2_PD1/1
  carr6_accumulator/1(Out_data) -> BitExtract11/1, BitExtract10/1
  Edge_deductor5/1(Out1) -> Carr2_PD1/2, Carr2_Accumulater4/2, Carr2_Accumulater3/2
  carr7_peak_dedector/2(pulse_1ms_out) -> Edge_deductor6/2(In2)
  Edge_deductor6/1(Out1) -> Carr3_PD2/2, Carr3_Accumulater5/2, Carr3_Accumulater6/2
  carr7_peak_dedector/1(Out_data) -> Carr3_PD2/1
  carr7_accumulator/1(Out_data) -> BitExtract13/1, BitExtract12/1
  BitExtract14/1 -> Carr3_Accumulater7/1
  BitExtract15/1 -> Carr3_Accumulater8/1
  carr8_peak_dedector/2(pulse_1ms_out) -> Edge_deductor7/2(In2)
  Edge_deductor7/1(Out1) -> Carr3_Accumulater8/2, Carr3_Accumulater7/2, Carr3_PD3/2
  carr8_peak_dedector/1(Out_data) -> Carr3_PD3/1
  carr8_accumulator/1(Out_data) -> BitExtract15/1, BitExtract14/1
  carr1_peak_dedector/1(Out_data) -> Carr1_PD/1

== system downlink_4c2t/DUT/DUC_SUMMER_PM ==
  note: I^2 + Q^2
  valid : Inport
  channel : Inport  Port=2
  "data " : Inport  Port=3
  pulse_1msec : Inport  Port=4
  Reg_busy_bit : Inport  Port=5
  Ant1_accumulator : Subsystem
  Ant1_peak_dedector : Subsystem
  Ant2_accumulator : Subsystem
  Ant2_peak_dedector : Subsystem
  BitExtract : DSPBAPrim/BitExtract  primtype=bitextract  nInputs=1  nOutputs=1  omode=Specify via dialog  otype=ufix(32)  scale=2^0  rndmethod=Unbiased  factor=1  satmethod=Symmetric  shift_vec=[0 1 2 -1]  value=0  inPortNames=[' '; ' ';]  outPortNames=[' ']  dspbaimage=dspba_prim.jpg  text=fprintf('..%d', value);  style=Optimised  visibilities=8+1024  version=20090407
  BitExtract1 : DSPBAPrim/BitExtract  primtype=bitextract  nInputs=1  nOutputs=1  omode=Specify via dialog  otype=ufix(32)  scale=2^0  rndmethod=Unbiased  factor=1  satmethod=Symmetric  shift_vec=[0 1 2 -1]  value=32  inPortNames=[' '; ' ';]  outPortNames=[' ']  dspbaimage=dspba_prim.jpg  text=fprintf('..%d', value);  style=Optimised  visibilities=8+1024  version=20090407
  BitExtract2 : DSPBAPrim/BitExtract  primtype=bitextract  nInputs=1  nOutputs=1  omode=Specify via dialog  otype=ufix(32)  scale=2^0  rndmethod=Unbiased  factor=1  satmethod=Symmetric  shift_vec=[0 1 2 -1]  value=0  inPortNames=[' '; ' ';]  outPortNames=[' ']  dspbaimage=dspba_prim.jpg  text=fprintf('..%d', value);  style=Optimised  visibilities=8+1024  version=20090407
  BitExtract3 : DSPBAPrim/BitExtract  primtype=bitextract  nInputs=1  nOutputs=1  omode=Specify via dialog  otype=ufix(32)  scale=2^0  rndmethod=Unbiased  factor=1  satmethod=Symmetric  shift_vec=[0 1 2 -1]  value=32  inPortNames=[' '; ' ';]  outPortNames=[' ']  dspbaimage=dspba_prim.jpg  text=fprintf('..%d', value);  style=Optimised  visibilities=8+1024  version=20090407
  Carr1_Accumulater1 : DSPBAModelBus/RegOut  reg_name=power_meter_param.summer_ant1_acc1_reg_addr  reg_rwmode=Read  reg_msb=31  reg_lsb=0  reg_desc=Description of what is stored in this register  reg_addr=9670  SampleTime=-1  version=20090407
  Carr1_Accumulater2 : DSPBAModelBus/RegOut  reg_name=power_meter_param.summer_ant1_acc2_reg_addr  reg_rwmode=Read  reg_msb=31  reg_lsb=0  reg_desc=Description of what is stored in this register  reg_addr=9671  SampleTime=-1  version=20090407
  Carr1_PD : DSPBAModelBus/RegOut  reg_name=power_meter_param.summer_ant1_pd_address  reg_rwmode=Read  reg_msb=31  reg_lsb=0  reg_desc=Description of what is stored in this register  reg_addr=9668  SampleTime=-1  version=20090407
  Carr2_Accumulater1 : DSPBAModelBus/RegOut  reg_name=power_meter_param.summer_ant2_acc1_reg_addr  reg_rwmode=Read  reg_msb=31  reg_lsb=0  reg_desc=Description of what is stored in this register  reg_addr=9672  SampleTime=-1  version=20090407
  Carr2_Accumulater2 : DSPBAModelBus/RegOut  reg_name=power_meter_param.summer_ant2_acc2_reg_addr  reg_rwmode=Read  reg_msb=31  reg_lsb=0  reg_desc=Description of what is stored in this register  reg_addr=9673  SampleTime=-1  version=20090407
  Carr2_PD : DSPBAModelBus/RegOut  reg_name=power_meter_param.summer_ant2_pd_address  reg_rwmode=Read  reg_msb=31  reg_lsb=0  reg_desc=Description of what is stored in this register  reg_addr=9669  SampleTime=-1  version=20090407
  Const : DSPBAPrim/Const  primtype=const  nInputs=0  nOutputs=1  omode=Inherit via internal rule  otype=sfix(16)  scale=2^-15  rndmethod=Unbiased  factor=1  satmethod=Symmetric  shift_vec=[0 1 2 -1]  value=0  inPortNames=['+'; '+';]  outPortNames=[' ']  dspbaimage=dspba_prim.jpg  text=fprintf('%s', num2str(value));  style=Optimised  visibilities=8 + 1024  floatPrecision=float32_m23  version=20120820
  Edge_deductor : Subsystem
  Edge_deductor1 : Subsystem
  Scale : DSPBABase/Scale  otype=sfix(16)  scale=2^-15  rndmethod=Unbiased  factor=1  satmethod=Symmetric  shift_vec=0  latency=6  wideSimulation=off  version=20130807
  Scale1 : DSPBABase/Scale  otype=sfix(16)  scale=2^-15  rndmethod=Unbiased  factor=1  satmethod=Symmetric  shift_vec=0  latency=6  wideSimulation=off  version=20130807
  Terminator1 : Terminator
  Terminator6 : Terminator
  carrier_separation : Subsystem
  wires:
  BitExtract3/1 -> Carr2_Accumulater2/1
  BitExtract2/1 -> Carr2_Accumulater1/1
  BitExtract1/1 -> Carr1_Accumulater2/1
  BitExtract/1 -> Carr1_Accumulater1/1
  Scale1/4 -> Terminator6/1
  carrier_separation/4(axc1_valid_out) -> Scale1/2
  carrier_separation/1(channel_out) -> Scale/3, Scale1/3
  carrier_separation/2(axc0_valid_out) -> Scale/2
  pulse_1msec/1 -> carrier_separation/4("1ms_pulse_in ")
  Scale/4 -> Terminator1/1
  "data "/1 -> carrier_separation/3("data ")
  channel/1 -> carrier_separation/2(channel)
  valid/1 -> carrier_separation/1(valid)
  carrier_separation/3("axc0_data_out ") -> Scale/1
  carrier_separation/5(axc1_data_out) -> Scale1/1
  Const/1 -> Scale/4, Scale1/4
  Scale/2 -> Ant1_accumulator/2(valid1), Ant1_peak_dedector/2(valid)
  Scale/1 -> Ant1_accumulator/1(data), Ant1_peak_dedector/1(data_in)
  Scale/3 -> Ant1_accumulator/3(channel1), Ant1_peak_dedector/3(channel)
  Scale1/1 -> Ant2_accumulator/1(data), Ant2_peak_dedector/1(data_in)
  Scale1/2 -> Ant2_accumulator/2(valid1), Ant2_peak_dedector/2(valid)
  Scale1/3 -> Ant2_accumulator/3(channel1), Ant2_peak_dedector/3(channel)
  carrier_separation/6(1ms_pulse_out) -> Ant2_peak_dedector/4(pulse_1ms), Ant1_accumulator/4(pulse_1ms), Ant1_peak_dedector/4(pulse_1ms), Ant2_accumulator/4(pulse_1ms)
  Ant1_peak_dedector/1(Out_data) -> Carr1_PD/1
  Edge_deductor/1(Out1) -> Carr1_Accumulater1/2, Carr1_Accumulater2/2, Carr1_PD/2
  Ant1_peak_dedector/2(pulse_1ms_out) -> Edge_deductor/2(In2)
  Ant1_accumulator/1(Out_data) -> BitExtract/1, BitExtract1/1
  Ant2_peak_dedector/2(pulse_1ms_out) -> Edge_deductor1/2(In2)
  Edge_deductor1/1(Out1) -> Carr2_PD/2, Carr2_Accumulater1/2, Carr2_Accumulater2/2
  Ant2_peak_dedector/1(Out_data) -> Carr2_PD/1
  Reg_busy_bit/1 -> Edge_deductor1/1(In1), Edge_deductor/1(In1)
  Ant2_accumulator/1(Out_data) -> BitExtract2/1, BitExtract3/1

== system downlink_4c2t/DUT/Downlink_ANT1_LB_rfp ==
  GPOut : DSPBAPrim/GPOut  primtype=gpout  nInputs=evalAionMaskParam(gcb,'value',1)  nOutputs=evalAionMaskParam(gcb,'value',1)  omode=Inherit via internal rule  otype=sfix(16)  scale=2^-15  rndmethod=Unbiased  factor=1  satmethod=Symmetric  shift_vec=[0 1 2 -1]  value=1  inPortNames=[' ' ' ' ' ' ' ' ' ' ' ' ' ' ' ' ' ' ' ' ' ' ' ' ' ' ' ' ' ' ' ' ' ' ' ' ' ' ' ' ' ' ' ' ' ' ' ' ' ' ' ' ' ' ' ' ' ' ' ' ' ' ' ' ' ' ' ' ' ']'  outPortNames=[' ' ' ' ' ' ' ' ' ' ' ' ' ' ' ' ' ' ' ' ' ' ' ' ' ' ' ' ' ' ' ' ' ' ' ' ' ' ' ' ' ' ' ' ' ' ' ' ' ' ' ' ' ' ' ' ' ' ' ' ' ' ' ' ' ' ' ' ' ']'  dspbaimage=dspba_prim.jpg  text=fprintf('GPOut');  style=Optimised  visibilities=1024  latencyCorrection=0  version=20090407
  SynthesisInfo : DSPBAPrim/SynthesisInfo  primtype=synthinfo  nInputs=0  nOutputs=0  omode=Inherit via internal rule  otype=sfix(16)  scale=2^-15  rndmethod=Truncate  factor=1  satmethod=Symmetric  shift_vec=[0 1 2 -1]  value=99  inPortNames=[' '; ' ';]  outPortNames=[' ']  dspbaimage=dspba_prim_ctrl.jpg  text=fprintf('Style=%s', style);  style=Scheduled  visibilities=2^15+2^17+2^18+2^19  constraintInUse=off  constraintRelation=>  constraintLimit=2  bitAccurate=off  version=20150220
  zero_idx1 : DSPBAPrim/Const  primtype=const  nInputs=0  nOutputs=1  omode=boolean  otype=ufix(1)  scale=0  rndmethod=Unbiased  factor=1  satmethod=Symmetric  shift_vec=[0 1 2 -1]  value=1  inPortNames=['+'; '+';]  outPortNames=[' ']  dspbaimage=dspba_prim.jpg  text=fprintf('%s', num2str(value));  style=Optimised  visibilities=8 + 1024  floatPrecision=float32_m23  version=20120820
  Out_RFP : Outport
  wires:
  GPOut/1 -> Out_RFP/1
  zero_idx1/1 -> GPOut/1

== system downlink_4c2t/DUT/Downlink_ANT1_RP_rfp ==
  GPOut : DSPBAPrim/GPOut  primtype=gpout  nInputs=evalAionMaskParam(gcb,'value',1)  nOutputs=evalAionMaskParam(gcb,'value',1)  omode=Inherit via internal rule  otype=sfix(16)  scale=2^-15  rndmethod=Unbiased  factor=1  satmethod=Symmetric  shift_vec=[0 1 2 -1]  value=1  inPortNames=[' ' ' ' ' ' ' ' ' ' ' ' ' ' ' ' ' ' ' ' ' ' ' ' ' ' ' ' ' ' ' ' ' ' ' ' ' ' ' ' ' ' ' ' ' ' ' ' ' ' ' ' ' ' ' ' ' ' ' ' ' ' ' ' ' ' ' ' ' ']'  outPortNames=[' ' ' ' ' ' ' ' ' ' ' ' ' ' ' ' ' ' ' ' ' ' ' ' ' ' ' ' ' ' ' ' ' ' ' ' ' ' ' ' ' ' ' ' ' ' ' ' ' ' ' ' ' ' ' ' ' ' ' ' ' ' ' ' ' ' ' ' ' ']'  dspbaimage=dspba_prim.jpg  text=fprintf('GPOut');  style=Optimised  visibilities=1024  latencyCorrection=0  version=20090407
  SynthesisInfo : DSPBAPrim/SynthesisInfo  primtype=synthinfo  nInputs=0  nOutputs=0  omode=Inherit via internal rule  otype=sfix(16)  scale=2^-15  rndmethod=Truncate  factor=1  satmethod=Symmetric  shift_vec=[0 1 2 -1]  value=99  inPortNames=[' '; ' ';]  outPortNames=[' ']  dspbaimage=dspba_prim_ctrl.jpg  text=fprintf('Style=%s', style);  style=Scheduled  visibilities=2^15+2^17+2^18+2^19  constraintInUse=off  constraintRelation=>  constraintLimit=2  bitAccurate=off  version=20150220
  zero_idx1 : DSPBAPrim/Const  primtype=const  nInputs=0  nOutputs=1  omode=boolean  otype=ufix(1)  scale=0  rndmethod=Unbiased  factor=1  satmethod=Symmetric  shift_vec=[0 1 2 -1]  value=1  inPortNames=['+'; '+';]  outPortNames=[' ']  dspbaimage=dspba_prim.jpg  text=fprintf('%s', num2str(value));  style=Optimised  visibilities=8 + 1024  floatPrecision=float32_m23  version=20120820
  Out_RFP : Outport
  wires:
  zero_idx1/1 -> GPOut/1
  GPOut/1 -> Out_RFP/1

== system downlink_4c2t/DUT/Gain_dpd_input ==
  a : Inport
  v : Inport  Port=2
  c : Inport  Port=3
  dpd1_gain_val : Inport  Port=4
  dpd2_gain_val : Inport  Port=5
  Subsystem : Subsystem
  Term : Terminator
  scale_gain : DSPBABase/Scale  otype=sfix(16 )  scale=2^-15  rndmethod=Unbiased  factor=1  satmethod=Symmetric  shift_vec=0  latency=7  wideSimulation=off  version=20090407
  zero_idx : DSPBAPrim/Const  primtype=const  nInputs=0  nOutputs=1  omode=Inherit via internal rule  otype=sfix(16)  scale=2^-15  rndmethod=Unbiased  factor=1  satmethod=Symmetric  shift_vec=[0 1 2 -1]  value=0  inPortNames=['+'; '+';]  outPortNames=[' ']  dspbaimage=dspba_prim.jpg  text=fprintf('%s', num2str(value));  style=Optimised  visibilities=8 + 1024  floatPrecision=float32_m23  version=20120820
  gain_real_out : Outport
  gain_v_out : Outport  Port=2
  gain_c_out : Outport  Port=3
  wires:
  dpd2_gain_val/1 -> Subsystem/5(dpd2_gain_val)
  dpd1_gain_val/1 -> Subsystem/4(dpd1_gain_val)
  scale_gain/3 -> gain_c_out/1
  scale_gain/2 -> gain_v_out/1
  scale_gain/1 -> gain_real_out/1
  Subsystem/3(gain_real_out) -> scale_gain/1
  Subsystem/2(gain_c_out) -> scale_gain/3
  Subsystem/1(gain_v_out) -> scale_gain/2
  zero_idx/1 -> scale_gain/4
  scale_gain/4 -> Term/1
  c/1 -> Subsystem/3(c)
  v/1 -> Subsystem/2(v)
  a/1 -> Subsystem/1(a)
